simulink model "QPSK"  (R2024a)
settings: Solver=ode45  StartTime=0.0  StopTime=1000  RelTol=1e-3  EnableMultiTasking=on
undefined symbols (not defined in the file): get
libraries: commdigbbndpm3 x3, commchan3 x1, commsink2 x1, commrandsrc3 x1
settings Model: Creator=Ammar  LastModifiedBy=Hoàng IRyS
settings SolverCC: AlgebraicLoopSolver=TrustRegion
settings DataIOCC: LimitDataPoints=on  SaveFormat=Array  SignalLoggingSaveFormat=ModelDataLogs  ReturnWorkspaceOutputs=off
settings OptimizationCC: ExpressionDepthLimit=2147483647  LifeSpan=inf
settings DebuggingCC: UnderspecifiedInitializationDetection=Classic  MergeDetectMultiDrivingBlocksExec=none  SolverPrmCheckMsg=warning  FcnCallInpInsideContextMsg=warning  UnconnectedInputMsg=warning  UnconnectedOutputMsg=warning  UnconnectedLineMsg=warning  StateNameClashWarn=warning  SFUnexpectedBacktrackingDiag=warning  SFNoUnconditionalDefaultTransitionDiag=warning  SFExecutionAtInitializationDiag=none  ArithmeticOperatorsInVariantConditions=warning
settings HardwareCC: ProdBitPerPointer=32  ProdBitPerSizeT=32  ProdBitPerPtrDiffT=32  ProdLargestAtomicFloat=None  ProdIntDivRoundTo=Undefined  ProdEndianess=Unspecified  ProdWordSize=32  ProdHWDeviceType=32-bit Generic
settings ModelReferenceCC: PropagateSignalLabelsOutOfModel=off
settings SFSimCC: SimUseLocalCustomCode=off  CustomCodeUndefinedFunction=UseInterfaceOnly
settings RTWCC: RTWUseLocalCustomCode=off  GPUComputeCapability=3.5
settings CodeAppCC: StateflowObjectComments=on
settings GRTTargetCC: TargetLangStandard=C89/C90 (ANSI)  CombineOutputUpdateFcns=off  GRTInterface=on
settings ConfigComp: CovMetricSettings=dw  CovSaveCumulativeToWorkspaceVar=on  CovSaveSingleToWorkspaceVar=on  CovExternalEMLEnable=off

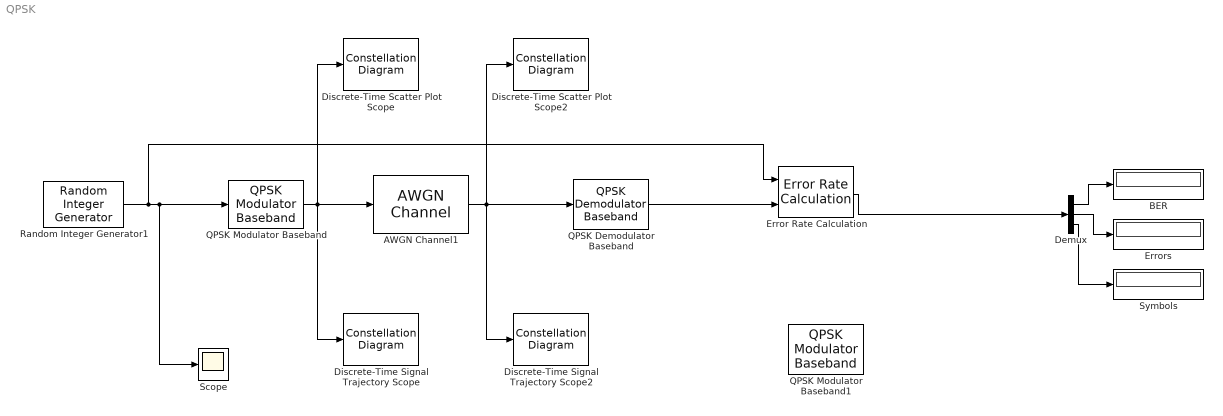
== system QPSK ==
  AWGN Channel1 : commchan3/AWGN Channel  LegacyMode=on  NoiseMethod="Signal to noise ratio  (SNR)"  noiseMode="Signal to noise ratio  (Eb/No)"  EbNo=-10  EsNo=6  SNR=3  BitsPerSymbol=2  SignalPower=1  SamplesPerSymbol=1  SymbolPeriod=1/1000  VarianceSource=Parameter  Variance=1  RandomStream=Global stream  Seed=67  SimulateUsing=Code generation
  BER : Display
  Demux : Demux  Outputs=3
  Discrete-Time Scatter Plot Scope : ConstellationDiagram  Tag=ScatterPlot  WindowPosition=[382.000000,84.000000,600.000000,600.000000,]  ScopeFrameLocation=window  FigPos=get(0,'defaultfigureposition');
  Discrete-Time Scatter Plot Scope2 : ConstellationDiagram  Tag=ScatterPlot  WindowPosition=[135.000000,-19.000000,600.000000,600.000000,]  ScopeFrameLocation=window  FigPos=get(0,'defaultfigureposition');
  Discrete-Time Signal Trajectory Scope : ConstellationDiagram  Tag=SignalTrajectory  WindowPosition=[449.000000,77.000000,560.000000,420.000000,]  ScopeFrameLocation=window  SamplesPerSymbol=8  SymbolsToDisplaySource=on  SymbolsToDisplay=40  Title=Signal Trajectory  XLimits=0.781352993211135  YLimits=0.781352993211135  ShowTrajectory=on  ColorFading=on  FigPos=get(0,'defaultfigureposition');
  Discrete-Time Signal Trajectory Scope2 : ConstellationDiagram  Tag=SignalTrajectory  WindowPosition=[886.000000,197.000000,560.000000,420.000000,]  ScopeFrameLocation=window  SamplesPerSymbol=8  SymbolsToDisplaySource=on  SymbolsToDisplay=40  Title=Signal Trajectory  XLimits=2  YLimits=2  ShowTrajectory=on  ColorFading=on  FigPos=get(0,'defaultfigureposition');
  Error Rate Calculation : commsink2/Error Rate Calculation  N=0  st_delay=0  cp_mode=Entire frame  subframe=[]  PMode=Port  WsName=ErrorVec  RsMode2=off  stop=off  numErr=100  maxBits=1e6
  Errors : Display
  QPSK Demodulator Baseband : commdigbbndpm3/QPSK Demodulator Baseband  OutType=Integer  DecType=Hard decision  VarSource=Dialog  Variance=1  Dec=Gray  Ph=pi/4  outDtype1=Inherit via internal rule  outDtype2=Inherit via internal rule  derotateFactorWordLen=16  derotateFactorDataTypeStr=Inherit: Same word length as input  derotateFactorLastDataTypeStr=Inherit: Same word length as input
  QPSK Modulator Baseband : commdigbbndpm3/QPSK Modulator Baseband  InType=Integer  Enc=Gray  Ph=pi/4  outDtype=double  outWordLen=16  outUDDataType=sfix(16)  outFracLenMode=Best precision  outFracLen=15  outDataTypeStr=double  outLastDataTypeStr=double
  QPSK Modulator Baseband1 : commdigbbndpm3/QPSK Modulator Baseband  InType=Integer  Enc=Gray  Ph=pi/4  outDtype=double  outWordLen=16  outUDDataType=sfix(16)  outFracLenMode=Best precision  outFracLen=15  outDataTypeStr=double  outLastDataTypeStr=double
  Random Integer Generator1 : commrandsrc3/Random Integer Generator  SetSize=4  SeedSource=Auto  Seed=67  SampleTime=1/1000  SamplesPerFrame=10  OutputDataType=double  SimulateUsing=Interpreted execution
  Scope : Scope
  Symbols : Display
  wires:
  Random Integer Generator1/1 -> Scope/1, QPSK Modulator Baseband/1, Error Rate Calculation/1
  Demux/1 -> BER/1
  Demux/2 -> Errors/1
  Demux/3 -> Symbols/1
  Error Rate Calculation/1 -> Demux/1
  QPSK Modulator Baseband/1 -> Discrete-Time Signal Trajectory Scope/1, Discrete-Time Scatter Plot Scope/1, AWGN Channel1/1
  AWGN Channel1/1 -> Discrete-Time Signal Trajectory Scope2/1, Discrete-Time Scatter Plot Scope2/1, QPSK Demodulator Baseband/1
  QPSK Demodulator Baseband/1 -> Error Rate Calculation/2
